simulink model "IdentificareFcnBuclaInterna"  (R2023b)
settings: Solver=FixedStepAuto  StartTime=0.0  StopTime=6  FixedStep=0.01  RelTol=1e-3
values from neighbouring files (symbols this model uses):
  k = 0.036    [CodDatepersonale.m]    (also in CodProiect.m = 0.035; untitled.m; untitled22.m = 0.035)
  k1 = 0.624    [CodDatepersonale.m]    (also in CodProiect.m = 0.654; untitled.m = 0.654; untitled22.m)
  k2 = -0.015    [CodDatepersonale.m]    (also in CodProiect.m; untitled.m; untitled22.m)
  k3 = -0.0006    [CodDatepersonale.m]    (also in CodProiect.m; untitled.m; untitled22.m)
  keta = 8*10^(-5)    (= 8e-05)    [CodDatepersonale.m]    (also in CodProiect.m; untitled.m; untitled22.m)
settings Model: Creator=Daniela  LastModifiedBy=Daniela

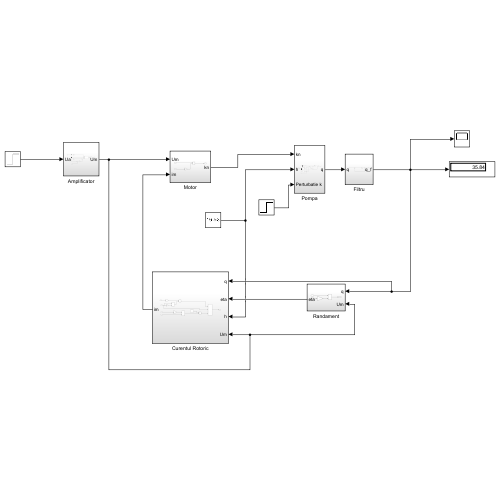
[thumbnail: Simulink's stored preview of the top-level diagram]
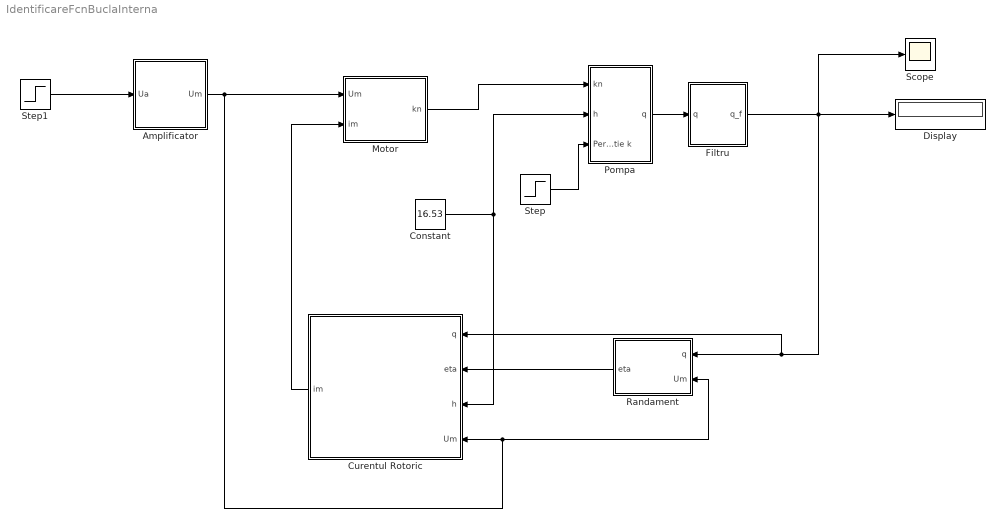
== system IdentificareFcnBuclaInterna ==
  Amplificator : Subsystem
  Constant : Constant  Value=16.53
  Curentul Rotoric : Subsystem
  Display : Display
  Filtru : Subsystem
  Motor : Subsystem
  Pompa : Subsystem
  Randament : Subsystem
  Scope : Scope
  Step : Step  Time=5000  After=0.0036  SampleTime=0
  Step1 : Step  Time=0  Before=5.6  After=6.1  SampleTime=0
  wires:
  Step/1 -> Pompa/3(Perturbatie k)
  Motor/1(kn) -> Pompa/1(kn)
  Step1/1 -> Amplificator/1(Ua)
  Randament/1(eta) -> Curentul Rotoric/2(eta)
  Curentul Rotoric/1(im) -> Motor/2(im)
  Pompa/1(q) -> Filtru/1(q)
  Constant/1 -> Pompa/2(h), Curentul Rotoric/3(h)
  Amplificator/1(Um) -> Motor/1(Um), Randament/2(Um), Curentul Rotoric/4(Um)
  Filtru/1(q_f) -> Display/1, Scope/1, Randament/1(q), Curentul Rotoric/1(q)

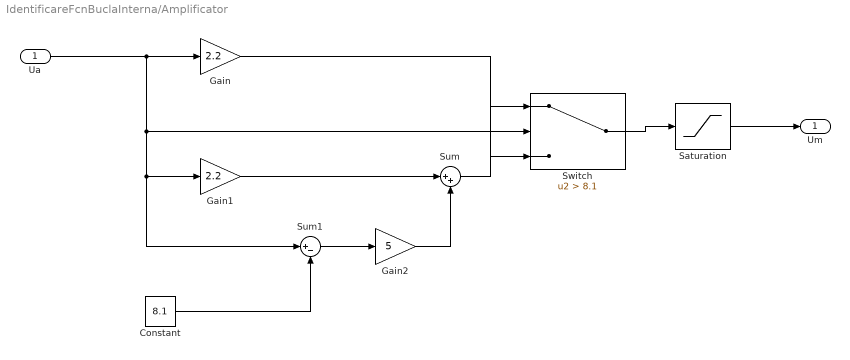
== system IdentificareFcnBuclaInterna/Amplificator ==
  Ua : Inport
  Constant : Constant  Value=8.1
  Gain : Gain  Gain=2.2
  Gain1 : Gain  Gain=2.2
  Gain2 : Gain  Gain=5
  Saturation : Saturate  UpperLimit=22  LowerLimit=0  ZeroCross=off
  Sum : Sum  Inputs=|++
  Sum1 : Sum  Inputs=|+-
  Switch : Switch  Criteria=u2 > Threshold  Threshold=8.1  SaturateOnIntegerOverflow=off  InputSameDT=off
  Um : Outport
  wires:
  Switch/1 -> Saturation/1
  Ua/1 -> Sum1/1, Gain1/1, Switch/2, Gain/1
  Constant/1 -> Sum1/2
  Sum1/1 -> Gain2/1
  Gain/1 -> Switch/3
  Sum/1 -> Switch/1
  Gain1/1 -> Sum/1
  Gain2/1 -> Sum/2
  Saturation/1 -> Um/1

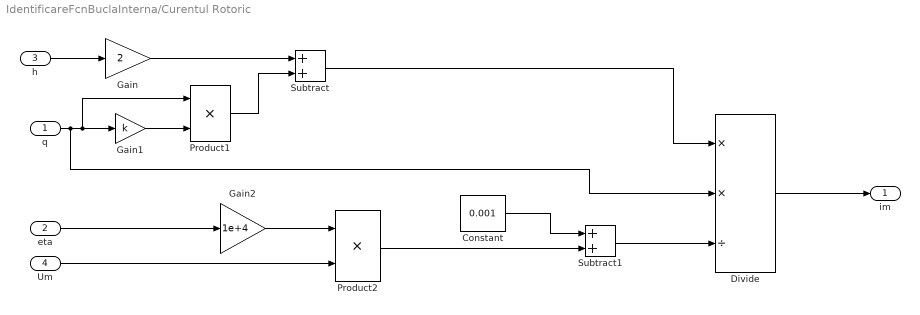
== system IdentificareFcnBuclaInterna/Curentul Rotoric ==
  q : Inport
  eta : Inport  Port=2
  h : Inport  Port=3
  Um : Inport  Port=4
  Constant : Constant  Value=0.001
  Divide : Product  Inputs=**/
  Gain : Gain  Gain=2
  Gain1 : Gain  Gain=k
  Gain2 : Gain  Gain=1e+4
  Product1 : Product
  Product2 : Product
  Subtract : Sum
  Subtract1 : Sum
  im : Outport
  wires:
  Product1/1 -> Subtract/2
  Um/1 -> Product2/2
  q/1 -> Gain1/1, Product1/1, Divide/2
  Subtract/1 -> Divide/1
  Divide/1 -> im/1
  Subtract1/1 -> Divide/3
  Gain2/1 -> Product2/1
  h/1 -> Gain/1
  Gain/1 -> Subtract/1
  Gain1/1 -> Product1/2
  eta/1 -> Gain2/1
  Product2/1 -> Subtract1/2
  Constant/1 -> Subtract1/1

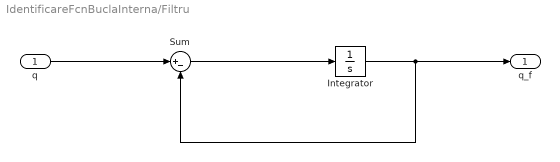
== system IdentificareFcnBuclaInterna/Filtru ==
  q : Inport
  Integrator : Integrator  InitialCondition=30.22
  Sum : Sum  Inputs=|+-
  q_f : Outport
  wires:
  Integrator/1 -> q_f/1, Sum/2
  q/1 -> Sum/1
  Sum/1 -> Integrator/1

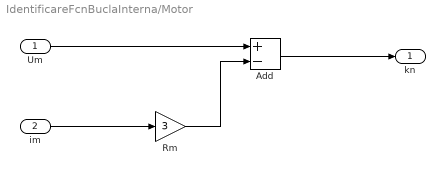
== system IdentificareFcnBuclaInterna/Motor ==
  Um : Inport
  im : Inport  Port=2
  Add : Sum  Inputs=+-
  Rm : Gain  Gain=3
  kn : Outport
  wires:
  im/1 -> Rm/1
  Add/1 -> kn/1
  Um/1 -> Add/1
  Rm/1 -> Add/2

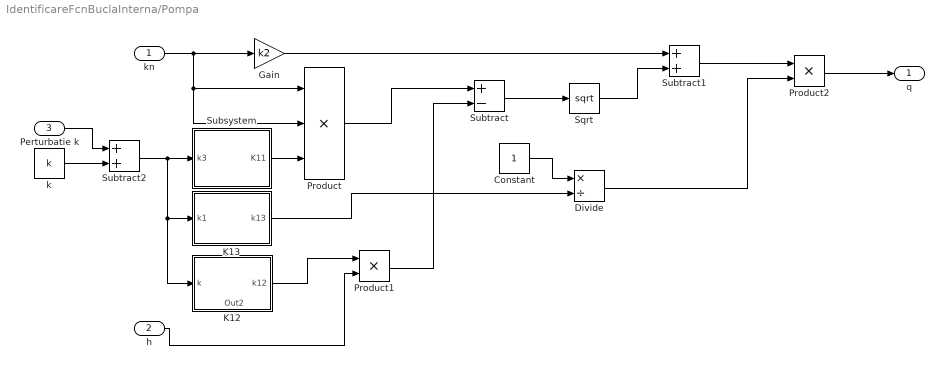
== system IdentificareFcnBuclaInterna/Pompa ==
  kn : Inport
  h : Inport  Port=2
  Perturbatie k : Inport  Port=3
  Constant : Constant
  Divide : Product  Inputs=*/
  Gain : Gain  Gain=k2
  K12 : Subsystem
      settings: PortSchema="{\"entries\":[{\"content\":{\"sides\":[{\"content\":{\"connectorIds\":[\"In1\"]},\"type\":\"ConnectorPlacement.EquallySpacedRectSide\",\"uuid\":\"47a044a6-8042-4edc-af6d-b4948b56e241\"},{\"content\":{\"connectorIds\":[\"Out1\"],\"side\":\"RIGHT\"},\"type\":\"ConnectorPlacement.EquallySpacedRectSide\",\"uuid\":\"2286c88f-0545-481f-8840-dcdd8ffee409\"},{\"content\":{\"side\":\"TOP\"},\"type\":\"ConnectorPlacement.EquallySpacedRectSide\",\"uuid\":\"70aa1e1a-3ba1-4bf2-81b0-86acd77959e1\"},{\"content\":{\"connectorIds\":[\"Out2\"],\"side\":\"BOTTOM\"},\"type\":\"ConnectorPlacement.EquallySpacedRectSide\",\"uuid\":\"a7cfce62-2dce-4250-a930-71fa11f65b45\"}]},\"type\":\"ConnectorPlacement.EquallySpacedConnector\",\"uuid\":\"18627665-8058-48fb-a085-cd52978710bb\"}],\"packageUris\":[\"http://schema.mathworks.com/mf0/Connector/R2020b\"],\"version\":\"1.0\"}"
  K13 : Subsystem
  Product : Product  Inputs=3
  Product1 : Product
  Product2 : Product
  Sqrt : Sqrt
  Subsystem : Subsystem
  Subtract : Sum  Inputs=+-
  Subtract1 : Sum
  Subtract2 : Sum
  k : Constant  Value=k
  q : Outport
  wires:
  Constant/1 -> Divide/1
  Subtract/1 -> Sqrt/1
  kn/1 -> Product/2, Product/1, Gain/1
  Product/1 -> Subtract/1
  Subsystem/1(K11) -> Product/3
  Sqrt/1 -> Subtract1/2
  Product2/1 -> q/1
  h/1 -> Product1/2
  Subtract2/1 -> Subsystem/1(k3), K12/1(k), K13/1(k1)
  Subtract1/1 -> Product2/1
  K13/1(k13) -> Divide/2
  Perturbatie k/1 -> Subtract2/1
  k/1 -> Subtract2/2
  Product1/1 -> Subtract/2
  Gain/1 -> Subtract1/1
  Divide/1 -> Product2/2
  K12/1(k12) -> Product1/1

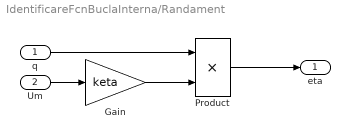
== system IdentificareFcnBuclaInterna/Randament ==
  q : Inport
  Um : Inport  Port=2
  Gain : Gain  Gain=keta
  Product : Product
  eta : Outport
  wires:
  Gain/1 -> Product/2
  Product/1 -> eta/1
  Um/1 -> Gain/1
  q/1 -> Product/1

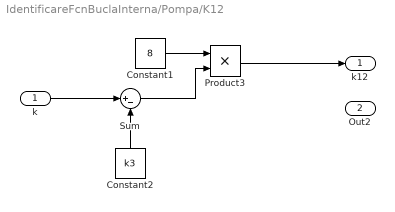
== system IdentificareFcnBuclaInterna/Pompa/K12 ==
  k : Inport
  Constant1 : Constant  Value=8
  Constant2 : Constant  Value=k3
  Product3 : Product
  Sum : Sum  Inputs=|+-
  k12 : Outport
  Out2 : Outport  Port=2
  wires:
  Sum/1 -> Product3/2
  k/1 -> Sum/1
  Constant1/1 -> Product3/1
  Product3/1 -> k12/1
  Constant2/1 -> Sum/2

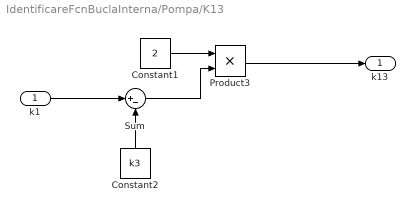
== system IdentificareFcnBuclaInterna/Pompa/K13 ==
  k1 : Inport
  Constant1 : Constant  Value=2
  Constant2 : Constant  Value=k3
  Product3 : Product
  Sum : Sum  Inputs=|+-
  k13 : Outport
  wires:
  Constant1/1 -> Product3/1
  Product3/1 -> k13/1
  Constant2/1 -> Sum/2
  k1/1 -> Sum/1
  Sum/1 -> Product3/2

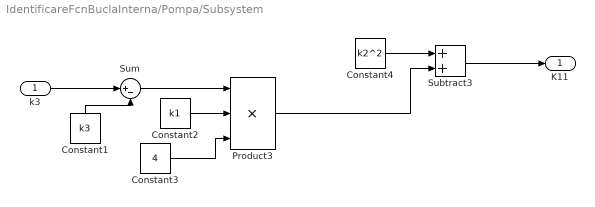
== system IdentificareFcnBuclaInterna/Pompa/Subsystem ==
  k3 : Inport
  Constant1 : Constant  Value=k3
  Constant2 : Constant  Value=k1
  Constant3 : Constant  Value=4
  Constant4 : Constant  Value=k2^2
  Product3 : Product  Inputs=3
  Subtract3 : Sum
  Sum : Sum  Inputs=|+-
  K11 : Outport
  wires:
  k3/1 -> Sum/1
  Subtract3/1 -> K11/1
  Product3/1 -> Subtract3/2
  Constant4/1 -> Subtract3/1
  Sum/1 -> Product3/1
  Constant1/1 -> Sum/2
  Constant3/1 -> Product3/3
  Constant2/1 -> Product3/2
